simulink model "motor_model_function"  (R2019b)
settings: Solver=VariableStepAuto  StartTime=0.0  StopTime=10.0  RelTol=1e-3
values from neighbouring files (symbols this model uses):
  Ts = evalin('base', 'Ts_motore')    [controllore_motore.m]    (also in phi_p_filter.m = evalin('base', 'Ts'); theta_p_filter.m = evalin('base', 'Ts'))
undefined symbols (not defined in the file or in its folder): controllore_motore, motor, sensitivity_arduino, Ts_motore
libraries: simulink x1
settings Model: Creator=miche  LastModifiedBy=miche

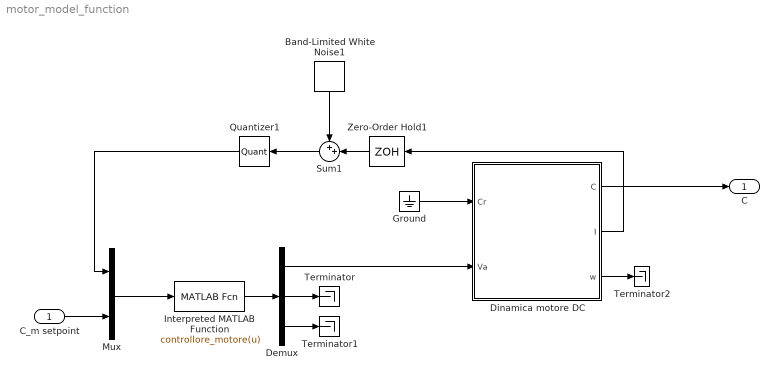
== system motor_model_function ==
  C_m setpoint : Inport  PortDimensions=1  SampleTime=Ts
  Band-Limited White Noise1 : simulink/Sources/Band-Limited White Noise  Cov=[0.0001]  Ts=0.001  seed=[23341]
  Demux : Demux  Outputs=3
  Dinamica motore DC : Subsystem
  Ground : Ground
  Interpreted MATLAB Function : MATLABFcn  MATLABFcn=controllore_motore(u)  OutputDimensions=3
  Mux : Mux  Inputs=2
      settings: DisplayOption=signals
  Quantizer1 : Quantizer  QuantizationInterval=1/sensitivity_arduino
  Sum1 : Sum  Inputs=++|
  Terminator : Terminator
  Terminator1 : Terminator
  Terminator2 : Terminator
  Zero-Order Hold1 : ZeroOrderHold  SampleTime=Ts_motore
  C : Outport  PortDimensions=1  SampleTime=Ts
  wires:
  Sum1/1 -> Quantizer1/1
  Demux/1 -> Dinamica motore DC/2(Va)
  Ground/1 -> Dinamica motore DC/1(Cr)
  Zero-Order Hold1/1 -> Sum1/2
  Band-Limited White Noise1/1 -> Sum1/1
  Dinamica motore DC/2(I) -> Zero-Order Hold1/1
  C_m setpoint/1 -> Mux/2
  Mux/1 -> Interpreted MATLAB Function/1
  Dinamica motore DC/1(C) -> C/1
  Quantizer1/1 -> Mux/1
  Interpreted MATLAB Function/1 -> Demux/1
  Demux/2 -> Terminator/1
  Demux/3 -> Terminator1/1
  Dinamica motore DC/3(w) -> Terminator2/1

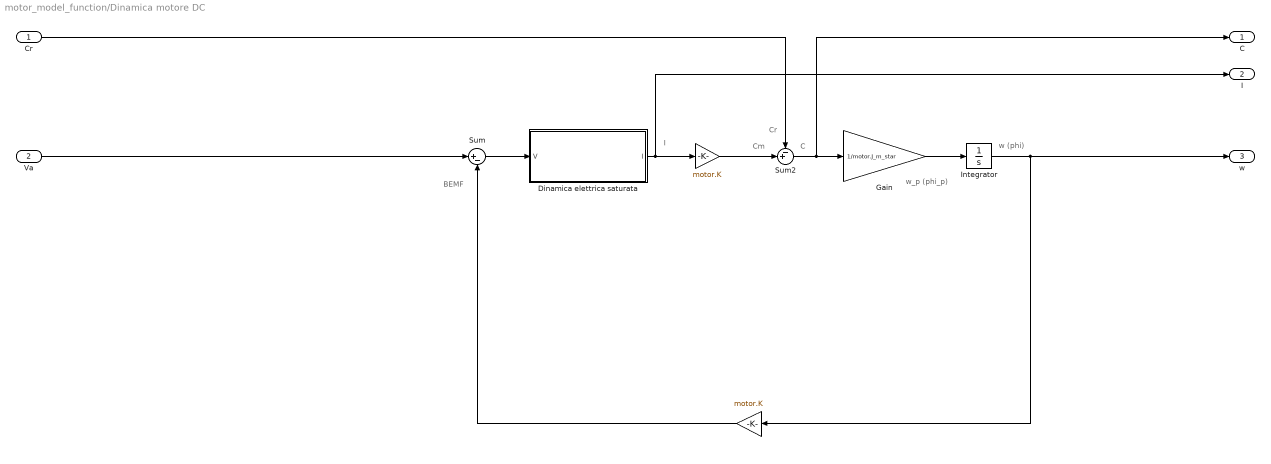
== system motor_model_function/Dinamica motore DC ==
  note: w (phi)
  note: C
  note: I
  note: Cm
  note: Cr
  note: w_p (phi_p)
  note: BEMF
  Cr : Inport
  Va : Inport  Port=2
  " " : Gain  Gain=motor.K
  " " : Gain  Gain=motor.K
  "Dinamica elettrica saturata " : Subsystem
  Gain : Gain  Gain=1/motor.J_m_star
  Integrator : Integrator
  Sum : Sum  Inputs=|+-
  Sum2 : Sum  Inputs=-+|
  C : Outport
  I : Outport  Port=2  PortDimensions=1
  w : Outport  Port=3
  wires:
  " "/1 -> Sum2/2
  Sum2/1 -> Gain/1, C/1
  Integrator/1 -> " "/1, w/1
  "Dinamica elettrica saturata "/1(I) -> I/1, " "/1
  Cr/1 -> Sum2/1
  " "/1 -> Sum/2
  Va/1 -> Sum/1
  Sum/1 -> "Dinamica elettrica saturata "/1(V)
  Gain/1 -> Integrator/1

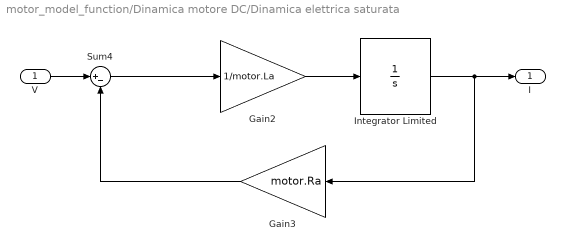
== system motor_model_function/Dinamica motore DC/Dinamica elettrica saturata  ==
  V : Inport
  Gain2 : Gain  Gain=1/motor.La
  Gain3 : Gain  Gain=motor.Ra
  Integrator Limited : Integrator  LimitOutput=on  UpperSaturationLimit=motor.Imax  LowerSaturationLimit=-motor.Imax
  Sum4 : Sum  Inputs=|+-
  I : Outport
  wires:
  Gain3/1 -> Sum4/2
  Sum4/1 -> Gain2/1
  Gain2/1 -> Integrator Limited/1
  Integrator Limited/1 -> I/1, Gain3/1
  V/1 -> Sum4/1
